simulink model "aerodynamic_model_V1"  (R2025b)
settings: Solver=ode4  StartTime=0.0  StopTime=sim_time  FixedStep=Ts  RelTol=1e-3
InitFcn:
  | % Run initial_main.m first to load Ad,As,Tq_prop,Tq_mass,...
values from neighbouring files (symbols this model uses):
  As = sys_sd.A    [initial_main.m]
  Bs = sys_sd.B    [initial_main.m]
  cg_m = eng.cg_m    [initial_main.m]
  Cs = sys_sd.C    [initial_main.m]
  Ds = sys_sd.D    [initial_main.m]
  DynamicsAndFlexibleStates_IC = Simulink.Bus.createMATLABStruct('DynamicsAndFlexibleStates')    [initial_main.m]
  e_thrust_cruise = eng.e_cruise    [initial_main.m]
  e_thrust_hover = eng.e_hover    [initial_main.m]
  eng_is_tilt = double(eng.is_tilt)    [initial_main.m]
  n_modes = size(Phi, 2)    [aeroelastic.m]    (also in initial_main.m = strips.n_modes)
  p_eng0_m = eng.p_eng_m    [initial_main.m]
  p_kink_m = eng.p_kink_m    [initial_main.m]
  polar_alpha_deg = polar.alpha_deg(:).'    [initial_main.m]
  polar_CD = polar.CD(:).'    [initial_main.m]
  polar_CDp = polar.CDp(:).'    [initial_main.m]
  polar_CL = polar.CL(:).'    [initial_main.m]
  polar_CM = polar.CM(:).'    [initial_main.m]
  R_sb = diag([-1, 1, -1])    [aeroelastic.m]    (also in initial_main.m = eng.R_sb)
  T_m2body = aeroelastic.node_kinematics(Phi, nodes).T_m2body    [initial_main.m]
  Tq_mass = load_maps.Tq_mass    [initial_main.m]
  Tq_prop = load_maps.Tq_prop    [initial_main.m]
  Ts = dt    (= 0.001)    [initial_main.m]
  U = hypot(38.69221536838454, 3.1651981735079)    [initial_main.m]
  v_tail_cant_rad = deg2rad(42)    [initial_main.m]
  W_mass_g = aeroelastic.gravity(nodes, 'g', g).W_mass    [initial_main.m]
  x0_structure = zeros(size(As, 1), 1)    [initial_main.m]
undefined symbols (not defined in the file or in its folder): Ad_v_tail_L, Ad_v_tail_R, Ad_wing_L, Ad_wing_R, alpha_du0_v_tail_L, alpha_du0_v_tail_R, alpha_du0_wing_L, alpha_du0_wing_R, Bd_v_tail_L, Bd_v_tail_R, Bd_wing_L, Bd_wing_R, c_over_2U_v_tail_L, c_over_2U_v_tail_R, c_over_2U_wing_L, c_over_2U_wing_R, Cd_v_tail_L, Cd_v_tail_R, Cd_wing_L, Cd_wing_R, cfd2d_ja, cfd2d_jl, cfd2d_kQ, cfd2d_kT, cfd2d_P1_CEF_X, cfd2d_P1_CEF_Y, cfd2d_P1_CEF_Z, cfd2d_P1_CEM_X, cfd2d_P1_CEM_Y, cfd2d_P1_CEM_Z, cfd2d_P5_CEF_X, cfd2d_P5_CEF_Y, cfd2d_P5_CEF_Z, cfd2d_P5_CEM_X, cfd2d_P5_CEM_Y, cfd2d_P5_CEM_Z, cfd3d_ja, cfd3d_jl, cfd3d_P2_CEF_X, cfd3d_P2_CEF_Y, cfd3d_P2_CEF_Z, cfd3d_P2_CEM_X, cfd3d_P2_CEM_Y, cfd3d_P2_CEM_Z, cfd3d_P6_CEF_X, cfd3d_P6_CEF_Y, cfd3d_P6_CEF_Z, cfd3d_P6_CEM_X, cfd3d_P6_CEM_Y, cfd3d_P6_CEM_Z, cfd3d_pitch, Dd_v_tail_L, Dd_v_tail_R, Dd_wing_L, Dd_wing_R, G_du_v_tail_L, G_du_v_tail_R, G_du_wing_L, G_du_wing_R, magnitude ... (+32)
(part 2 of 2)

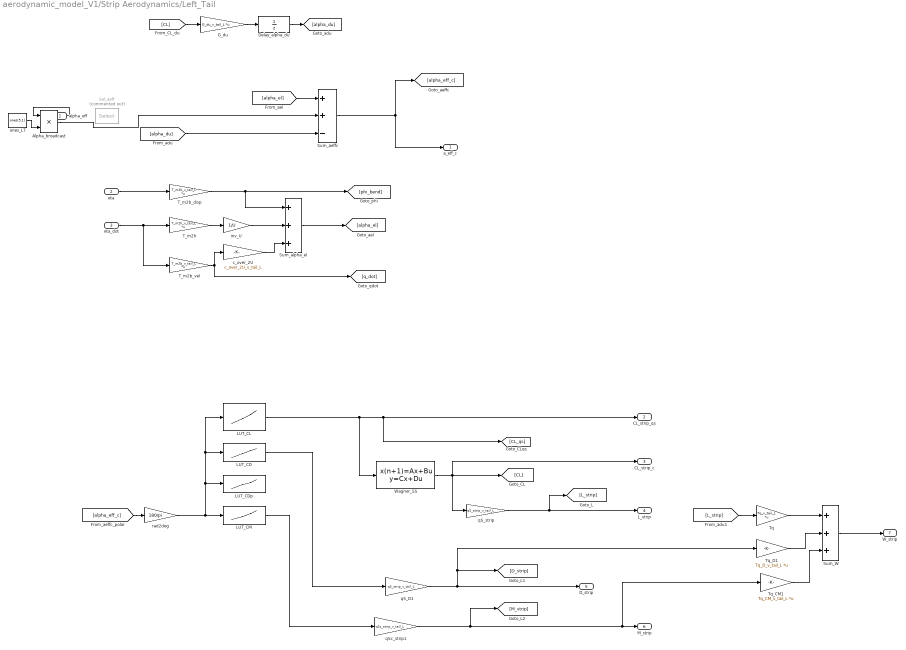
== system aerodynamic_model_V1/Strip Aerodynamics/Left_Tail ==
  alpha_eff : Inport  PortDimensions=1
  eta : Inport  Port=2  PortDimensions=21
  eta_dot : Inport  Port=3  PortDimensions=21
  Alpha_broadcast : Product  Inputs=**
  Delay_alpha_du : UnitDelay  InitialCondition=alpha_du0_v_tail_L  SampleTime=Ts  HasFrameUpgradeWarning=on
  G_du : Gain  Gain=G_du_v_tail_L  Multiplication=Matrix(K*u)
  LUT_CD : Lookup_n-D  NumberOfTableDimensions=1  BreakpointsForDimension1=polar_alpha_deg  BreakpointsForDimension3=[5, 7]  Table=polar_CD  ExtrapMethod=Clip  InternalRulePriority=Speed  RndMeth=Simplest
  LUT_CDp : Lookup_n-D  NumberOfTableDimensions=1  BreakpointsForDimension1=polar_alpha_deg  BreakpointsForDimension3=[5, 7]  Table=polar_CDp  ExtrapMethod=Clip  InternalRulePriority=Speed  RndMeth=Simplest
  LUT_CL : Lookup_n-D  NumberOfTableDimensions=1  BreakpointsForDimension1=polar_alpha_deg  BreakpointsForDimension3=[5, 7]  Table=polar_CL  ExtrapMethod=Clip  InternalRulePriority=Speed  RndMeth=Simplest
  LUT_CM : Lookup_n-D  NumberOfTableDimensions=1  BreakpointsForDimension1=polar_alpha_deg  BreakpointsForDimension3=[5, 7]  Table=polar_CM  ExtrapMethod=Clip  InternalRulePriority=Speed  RndMeth=Simplest
  Sel_aeff : Selector  Commented=on  InputPortWidth=n_strip  IndexOptions=Select all  Indices=idx_v_tail_L  OutputSizes=n_strip_v_tail_L
  Sum_W : Sum  Inputs=+++
  Sum_aeffc : Sum  Inputs=++-
  Sum_alpha_el : Sum  Inputs=+++
  T_m2b_disp : Gain  Gain=T_m2b_v_tail_L  Multiplication=Matrix(K*u)
  T_m2b_vel : Gain  Gain=T_m2b_v_tail_L  Multiplication=Matrix(K*u)
  T_m2h : Gain  Gain=T_m2h_v_tail_L  Multiplication=Matrix(K*u)
  Tq : Gain  Gain=Tq_v_tail_L  Multiplication=Matrix(K*u)
  Tq_CM1 : Gain  Gain=Tq_CM_v_tail_L  Multiplication=Matrix(K*u)
  Tq_D1 : Gain  Gain=Tq_D_v_tail_L  Multiplication=Matrix(K*u)
  Wagner_SS : DiscreteStateSpace  A=Ad_v_tail_L  B=Bd_v_tail_L  C=Cd_v_tail_L  D=Dd_v_tail_L  InitialCondition=x0_wagner_v_tail_L  SampleTime=Ts
  c_over_2U : Gain  Gain=c_over_2U_v_tail_L
  inv_U : Gain  Gain=1/U
  ones_LT : Constant  Value=ones(5,1)
  qS_D1 : Gain  Gain=qS_strip_v_tail_L
  qS_strip : Gain  Gain=qS_strip_v_tail_L
  qSc_strip1 : Gain  Gain=qSc_strip_v_tail_L
  rad2deg : Gain  Gain=180/pi
  a_eff_c : Outport
  CL_strip_qs : Outport  Port=2
  CL_strip_c : Outport  Port=3
  L_strip : Outport  Port=4
  D_strip : Outport  Port=5
  M_strip : Outport  Port=6
  W_strip : Outport  Port=7
  wires:
  rad2deg/1 -> LUT_CL/1, LUT_CD/1, LUT_CDp/1, LUT_CM/1
  Wagner_SS/1 -> [CL], CL_strip_c/1, qS_strip/1
  eta/1 -> T_m2b_disp/1
  Delay_alpha_du/1 -> [alpha_du]
  qS_strip/1 -> L_strip/1, [L_strip]
  LUT_CL/1 -> CL_strip_qs/1, [CL_qs], Wagner_SS/1
  T_m2b_vel/1 -> c_over_2U/1, [q_dot]
  inv_U/1 -> Sum_alpha_el/2
  T_m2b_disp/1 -> Sum_alpha_el/1, [phi_bend]
  G_du/1 -> Delay_alpha_du/1
  c_over_2U/1 -> Sum_alpha_el/3
  Sum_alpha_el/1 -> [alpha_el]
  Sum_aeffc/1 -> a_eff_c/1, [alpha_eff_c]
  [alpha_eff_c] -> rad2deg/1
  T_m2h/1 -> inv_U/1
  eta_dot/1 -> T_m2b_vel/1, T_m2h/1
  LUT_CD/1 -> qS_D1/1
  LUT_CM/1 -> qSc_strip1/1
  [CL] -> G_du/1
  [alpha_el] -> Sum_aeffc/1
  [alpha_du] -> Sum_aeffc/3
  qS_D1/1 -> Tq_D1/1, [D_strip], D_strip/1
  qSc_strip1/1 -> M_strip/1, Tq_CM1/1, [M_strip]
  [L_strip] -> Tq/1
  Tq/1 -> Sum_W/1
  Tq_D1/1 -> Sum_W/2
  Tq_CM1/1 -> Sum_W/3
  Sum_W/1 -> W_strip/1
  alpha_eff/1 -> Alpha_broadcast/1
  ones_LT/1 -> Alpha_broadcast/2
  Alpha_broadcast/1 -> Sum_aeffc/2

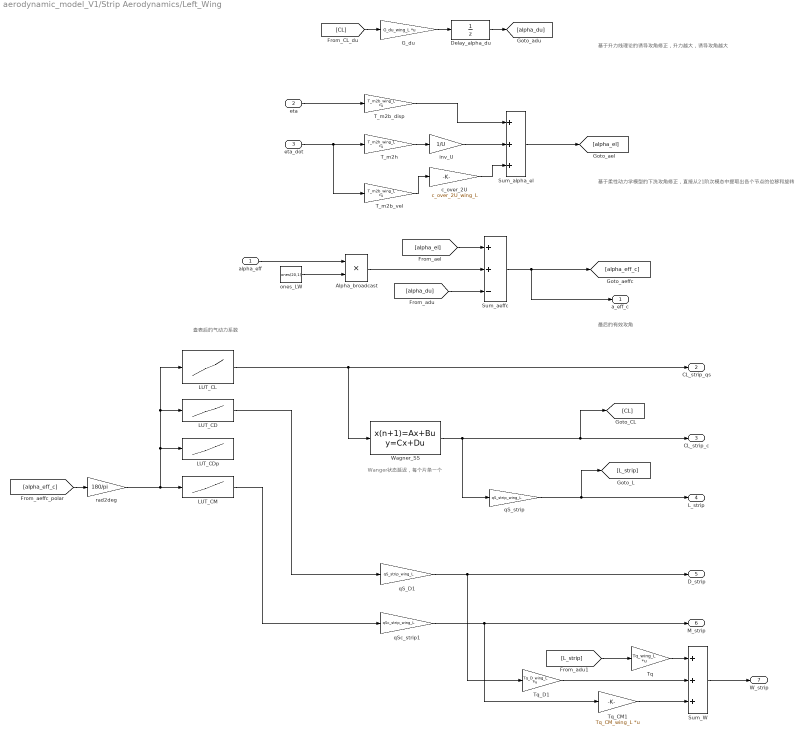
== system aerodynamic_model_V1/Strip Aerodynamics/Left_Wing ==
  note: 基于升力线理论的诱导攻角修正，升力越大，诱导攻角越大
  note: 基于柔性动力学模型的下洗攻角修正，直接从21阶次模态中提取出各个节点的位移和旋转
  note: 最后的有效攻角
  note: 查表后的气动力系数
  note: Wanger状态延迟，每个片条一个
  alpha_eff : Inport  PortDimensions=1
  eta : Inport  Port=2  PortDimensions=21
  eta_dot : Inport  Port=3  PortDimensions=21
  Alpha_broadcast : Product  Inputs=**
  Delay_alpha_du : UnitDelay  InitialCondition=alpha_du0_wing_L  SampleTime=Ts  HasFrameUpgradeWarning=on
  G_du : Gain  Gain=G_du_wing_L  Multiplication=Matrix(K*u)
  LUT_CD : Lookup_n-D  NumberOfTableDimensions=1  BreakpointsForDimension1=polar_alpha_deg  BreakpointsForDimension3=[5, 7]  Table=polar_CD  ExtrapMethod=Clip  InternalRulePriority=Speed  RndMeth=Simplest
  LUT_CDp : Lookup_n-D  NumberOfTableDimensions=1  BreakpointsForDimension1=polar_alpha_deg  BreakpointsForDimension3=[5, 7]  Table=polar_CDp  ExtrapMethod=Clip  InternalRulePriority=Speed  RndMeth=Simplest
  LUT_CL : Lookup_n-D  NumberOfTableDimensions=1  BreakpointsForDimension1=polar_alpha_deg  BreakpointsForDimension3=[5, 7]  Table=polar_CL  ExtrapMethod=Clip  InternalRulePriority=Speed  RndMeth=Simplest
  LUT_CM : Lookup_n-D  NumberOfTableDimensions=1  BreakpointsForDimension1=polar_alpha_deg  BreakpointsForDimension3=[5, 7]  Table=polar_CM  ExtrapMethod=Clip  InternalRulePriority=Speed  RndMeth=Simplest
  Sum_W : Sum  Inputs=+++
  Sum_aeffc : Sum  Inputs=++-
  Sum_alpha_el : Sum  Inputs=+++
  T_m2b_disp : Gain  Gain=T_m2b_wing_L  Multiplication=Matrix(K*u)
  T_m2b_vel : Gain  Gain=T_m2b_wing_L  Multiplication=Matrix(K*u)
  T_m2h : Gain  Gain=T_m2h_wing_L  Multiplication=Matrix(K*u)
  Tq : Gain  Gain=Tq_wing_L  Multiplication=Matrix(K*u)
  Tq_CM1 : Gain  Gain=Tq_CM_wing_L  Multiplication=Matrix(K*u)
  Tq_D1 : Gain  Gain=Tq_D_wing_L  Multiplication=Matrix(K*u)
  Wagner_SS : DiscreteStateSpace  A=Ad_wing_L  B=Bd_wing_L  C=Cd_wing_L  D=Dd_wing_L  InitialCondition=x0_wagner_wing_L  SampleTime=Ts
  c_over_2U : Gain  Gain=c_over_2U_wing_L
  inv_U : Gain  Gain=1/U
  ones_LW : Constant  Value=ones(20,1)
  qS_D1 : Gain  Gain=qS_strip_wing_L
  qS_strip : Gain  Gain=qS_strip_wing_L
  qSc_strip1 : Gain  Gain=qSc_strip_wing_L
  rad2deg : Gain  Gain=180/pi
  a_eff_c : Outport
  CL_strip_qs : Outport  Port=2
  CL_strip_c : Outport  Port=3
  L_strip : Outport  Port=4
  D_strip : Outport  Port=5
  M_strip : Outport  Port=6
  W_strip : Outport  Port=7
  wires:
  rad2deg/1 -> LUT_CL/1, LUT_CD/1, LUT_CDp/1, LUT_CM/1
  Wagner_SS/1 -> [CL], CL_strip_c/1, qS_strip/1
  eta/1 -> T_m2b_disp/1
  Delay_alpha_du/1 -> [alpha_du]
  qS_strip/1 -> L_strip/1, [L_strip]
  LUT_CL/1 -> CL_strip_qs/1, Wagner_SS/1
  T_m2b_vel/1 -> c_over_2U/1
  inv_U/1 -> Sum_alpha_el/2
  T_m2b_disp/1 -> Sum_alpha_el/1
  G_du/1 -> Delay_alpha_du/1
  c_over_2U/1 -> Sum_alpha_el/3
  Sum_alpha_el/1 -> [alpha_el]
  Sum_aeffc/1 -> a_eff_c/1, [alpha_eff_c]
  [alpha_eff_c] -> rad2deg/1
  T_m2h/1 -> inv_U/1
  eta_dot/1 -> T_m2b_vel/1, T_m2h/1
  LUT_CD/1 -> qS_D1/1
  LUT_CM/1 -> qSc_strip1/1
  [CL] -> G_du/1
  [alpha_el] -> Sum_aeffc/1
  [alpha_du] -> Sum_aeffc/3
  qS_D1/1 -> D_strip/1, Tq_D1/1
  qSc_strip1/1 -> M_strip/1, Tq_CM1/1
  [L_strip] -> Tq/1
  Tq/1 -> Sum_W/1
  Tq_D1/1 -> Sum_W/2
  Tq_CM1/1 -> Sum_W/3
  Sum_W/1 -> W_strip/1
  alpha_eff/1 -> Alpha_broadcast/1
  ones_LW/1 -> Alpha_broadcast/2
  Alpha_broadcast/1 -> Sum_aeffc/2

== system aerodynamic_model_V1/Strip Aerodynamics/Local_Alphas ==
  V_b : Inport  PortDimensions=3
  cant : Inport  Port=2  PortDimensions=1
  fcn : MATLAB Function  TreatAsAtomicUnit=on
  a_wr : Outport
  a_wl : Outport  Port=2
  a_tr : Outport  Port=3
  a_tl : Outport  Port=4
  wires:
  V_b/1 -> fcn/1(V_b)
  cant/1 -> fcn/2(cant)
  fcn/1(a_wr) -> a_wr/1
  fcn/2(a_wl) -> a_wl/1
  fcn/3(a_tr) -> a_tr/1
  fcn/4(a_tl) -> a_tl/1

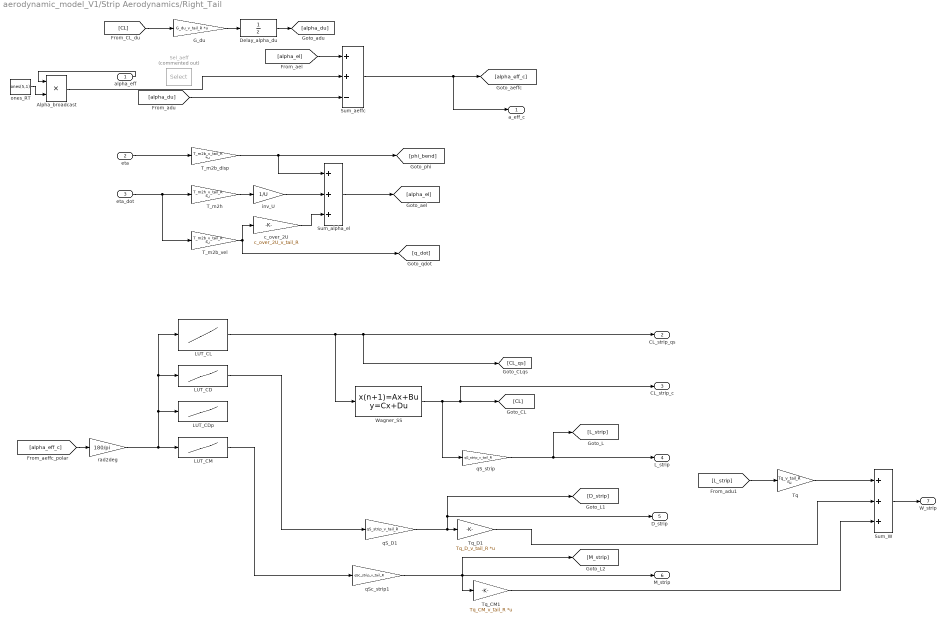
== system aerodynamic_model_V1/Strip Aerodynamics/Right_Tail ==
  alpha_eff : Inport  PortDimensions=1
  eta : Inport  Port=2  PortDimensions=21
  eta_dot : Inport  Port=3  PortDimensions=21
  Alpha_broadcast : Product  Inputs=**
  Delay_alpha_du : UnitDelay  InitialCondition=alpha_du0_v_tail_R  SampleTime=Ts  HasFrameUpgradeWarning=on
  G_du : Gain  Gain=G_du_v_tail_R  Multiplication=Matrix(K*u)
  LUT_CD : Lookup_n-D  NumberOfTableDimensions=1  BreakpointsForDimension1=polar_alpha_deg  BreakpointsForDimension3=[5, 7]  Table=polar_CD  ExtrapMethod=Clip  InternalRulePriority=Speed  RndMeth=Simplest
  LUT_CDp : Lookup_n-D  NumberOfTableDimensions=1  BreakpointsForDimension1=polar_alpha_deg  BreakpointsForDimension3=[5, 7]  Table=polar_CDp  ExtrapMethod=Clip  InternalRulePriority=Speed  RndMeth=Simplest
  LUT_CL : Lookup_n-D  NumberOfTableDimensions=1  BreakpointsForDimension1=polar_alpha_deg  BreakpointsForDimension3=[5, 7]  Table=polar_CL  ExtrapMethod=Clip  InternalRulePriority=Speed  RndMeth=Simplest
  LUT_CM : Lookup_n-D  NumberOfTableDimensions=1  BreakpointsForDimension1=polar_alpha_deg  BreakpointsForDimension3=[5, 7]  Table=polar_CM  ExtrapMethod=Clip  InternalRulePriority=Speed  RndMeth=Simplest
  Sel_aeff : Selector  Commented=on  InputPortWidth=n_strip  IndexOptions=Select all  Indices=idx_v_tail_R  OutputSizes=n_strip_v_tail_R
  Sum_W : Sum  Inputs=+++
  Sum_aeffc : Sum  Inputs=++-
  Sum_alpha_el : Sum  Inputs=+++
  T_m2b_disp : Gain  Gain=T_m2b_v_tail_R  Multiplication=Matrix(K*u)
  T_m2b_vel : Gain  Gain=T_m2b_v_tail_R  Multiplication=Matrix(K*u)
  T_m2h : Gain  Gain=T_m2h_v_tail_R  Multiplication=Matrix(K*u)
  Tq : Gain  Gain=Tq_v_tail_R  Multiplication=Matrix(K*u)
  Tq_CM1 : Gain  Gain=Tq_CM_v_tail_R  Multiplication=Matrix(K*u)
  Tq_D1 : Gain  Gain=Tq_D_v_tail_R  Multiplication=Matrix(K*u)
  Wagner_SS : DiscreteStateSpace  A=Ad_v_tail_R  B=Bd_v_tail_R  C=Cd_v_tail_R  D=Dd_v_tail_R  InitialCondition=x0_wagner_v_tail_R  SampleTime=Ts
  c_over_2U : Gain  Gain=c_over_2U_v_tail_R
  inv_U : Gain  Gain=1/U
  ones_RT : Constant  Value=ones(5,1)
  qS_D1 : Gain  Gain=qS_strip_v_tail_R
  qS_strip : Gain  Gain=qS_strip_v_tail_R
  qSc_strip1 : Gain  Gain=qSc_strip_v_tail_R
  rad2deg : Gain  Gain=180/pi
  a_eff_c : Outport
  CL_strip_qs : Outport  Port=2
  CL_strip_c : Outport  Port=3
  L_strip : Outport  Port=4
  D_strip : Outport  Port=5
  M_strip : Outport  Port=6
  W_strip : Outport  Port=7
  wires:
  rad2deg/1 -> LUT_CL/1, LUT_CD/1, LUT_CDp/1, LUT_CM/1
  Wagner_SS/1 -> CL_strip_c/1, [CL], qS_strip/1
  eta/1 -> T_m2b_disp/1
  Delay_alpha_du/1 -> [alpha_du]
  qS_strip/1 -> L_strip/1, [L_strip]
  LUT_CL/1 -> CL_strip_qs/1, [CL_qs], Wagner_SS/1
  T_m2b_vel/1 -> c_over_2U/1, [q_dot]
  inv_U/1 -> Sum_alpha_el/2
  T_m2b_disp/1 -> Sum_alpha_el/1, [phi_bend]
  G_du/1 -> Delay_alpha_du/1
  c_over_2U/1 -> Sum_alpha_el/3
  Sum_alpha_el/1 -> [alpha_el]
  Sum_aeffc/1 -> a_eff_c/1, [alpha_eff_c]
  [alpha_eff_c] -> rad2deg/1
  T_m2h/1 -> inv_U/1
  eta_dot/1 -> T_m2b_vel/1, T_m2h/1
  LUT_CD/1 -> qS_D1/1
  LUT_CM/1 -> qSc_strip1/1
  [CL] -> G_du/1
  [alpha_el] -> Sum_aeffc/1
  [alpha_du] -> Sum_aeffc/3
  qS_D1/1 -> D_strip/1, [D_strip], Tq_D1/1
  qSc_strip1/1 -> [M_strip], M_strip/1, Tq_CM1/1
  [L_strip] -> Tq/1
  Tq/1 -> Sum_W/1
  Tq_D1/1 -> Sum_W/2
  Tq_CM1/1 -> Sum_W/3
  Sum_W/1 -> W_strip/1
  alpha_eff/1 -> Alpha_broadcast/1
  ones_RT/1 -> Alpha_broadcast/2
  Alpha_broadcast/1 -> Sum_aeffc/2

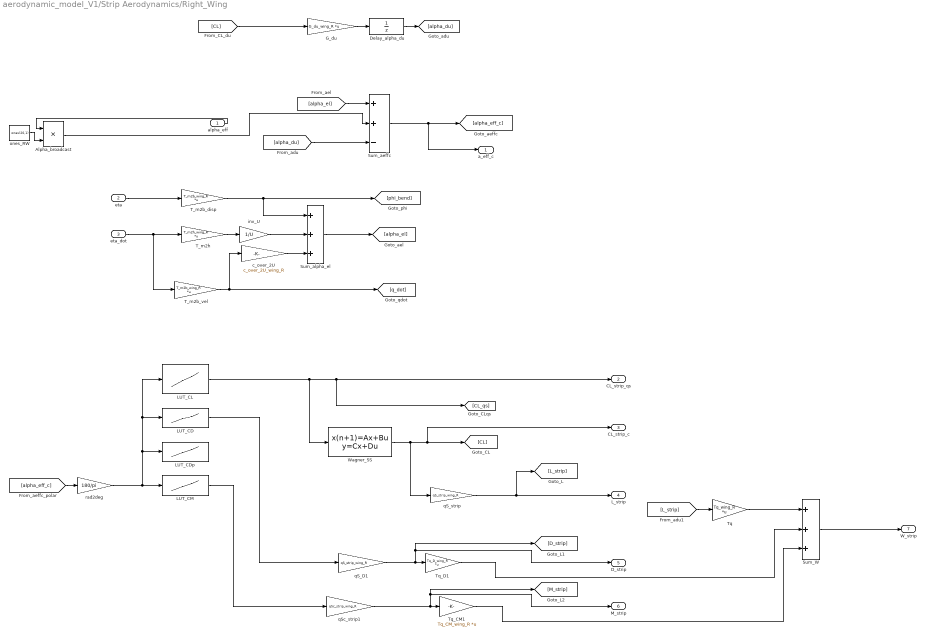
== system aerodynamic_model_V1/Strip Aerodynamics/Right_Wing ==
  alpha_eff : Inport  PortDimensions=1
  eta : Inport  Port=2  PortDimensions=21
  eta_dot : Inport  Port=3  PortDimensions=21
  Alpha_broadcast : Product  Inputs=**
  Delay_alpha_du : UnitDelay  InitialCondition=alpha_du0_wing_R  SampleTime=Ts  HasFrameUpgradeWarning=on
  G_du : Gain  Gain=G_du_wing_R  Multiplication=Matrix(K*u)
  LUT_CD : Lookup_n-D  NumberOfTableDimensions=1  BreakpointsForDimension1=polar_alpha_deg  BreakpointsForDimension3=[5, 7]  Table=polar_CD  ExtrapMethod=Clip  InternalRulePriority=Speed  RndMeth=Simplest
  LUT_CDp : Lookup_n-D  NumberOfTableDimensions=1  BreakpointsForDimension1=polar_alpha_deg  BreakpointsForDimension3=[5, 7]  Table=polar_CDp  ExtrapMethod=Clip  InternalRulePriority=Speed  RndMeth=Simplest
  LUT_CL : Lookup_n-D  NumberOfTableDimensions=1  BreakpointsForDimension1=polar_alpha_deg  BreakpointsForDimension3=[5, 7]  Table=polar_CL  ExtrapMethod=Clip  InternalRulePriority=Speed  RndMeth=Simplest
  LUT_CM : Lookup_n-D  NumberOfTableDimensions=1  BreakpointsForDimension1=polar_alpha_deg  BreakpointsForDimension3=[5, 7]  Table=polar_CM  ExtrapMethod=Clip  InternalRulePriority=Speed  RndMeth=Simplest
  Sum_W : Sum  Inputs=+++
  Sum_aeffc : Sum  Inputs=++-
  Sum_alpha_el : Sum  Inputs=+++
  T_m2b_disp : Gain  Gain=T_m2b_wing_R  Multiplication=Matrix(K*u)
  T_m2b_vel : Gain  Gain=T_m2b_wing_R  Multiplication=Matrix(K*u)
  T_m2h : Gain  Gain=T_m2h_wing_R  Multiplication=Matrix(K*u)
  Tq : Gain  Gain=Tq_wing_R  Multiplication=Matrix(K*u)
  Tq_CM1 : Gain  Gain=Tq_CM_wing_R  Multiplication=Matrix(K*u)
  Tq_D1 : Gain  Gain=Tq_D_wing_R  Multiplication=Matrix(K*u)
  Wagner_SS : DiscreteStateSpace  A=Ad_wing_R  B=Bd_wing_R  C=Cd_wing_R  D=Dd_wing_R  InitialCondition=x0_wagner_wing_R  SampleTime=Ts
  c_over_2U : Gain  Gain=c_over_2U_wing_R
  inv_U : Gain  Gain=1/U
  ones_RW : Constant  Value=ones(20,1)
  qS_D1 : Gain  Gain=qS_strip_wing_R
  qS_strip : Gain  Gain=qS_strip_wing_R
  qSc_strip1 : Gain  Gain=qSc_strip_wing_R
  rad2deg : Gain  Gain=180/pi
  a_eff_c : Outport
  CL_strip_qs : Outport  Port=2
  CL_strip_c : Outport  Port=3
  L_strip : Outport  Port=4
  D_strip : Outport  Port=5
  M_strip : Outport  Port=6
  W_strip : Outport  Port=7
  wires:
  rad2deg/1 -> LUT_CL/1, LUT_CD/1, LUT_CDp/1, LUT_CM/1
  Wagner_SS/1 -> CL_strip_c/1, [CL], qS_strip/1
  eta/1 -> T_m2b_disp/1
  Delay_alpha_du/1 -> [alpha_du]
  qS_strip/1 -> L_strip/1, [L_strip]
  LUT_CL/1 -> CL_strip_qs/1, [CL_qs], Wagner_SS/1
  T_m2b_vel/1 -> c_over_2U/1, [q_dot]
  inv_U/1 -> Sum_alpha_el/2
  T_m2b_disp/1 -> Sum_alpha_el/1, [phi_bend]
  G_du/1 -> Delay_alpha_du/1
  c_over_2U/1 -> Sum_alpha_el/3
  Sum_alpha_el/1 -> [alpha_el]
  Sum_aeffc/1 -> a_eff_c/1, [alpha_eff_c]
  [alpha_eff_c] -> rad2deg/1
  T_m2h/1 -> inv_U/1
  eta_dot/1 -> T_m2b_vel/1, T_m2h/1
  LUT_CD/1 -> qS_D1/1
  LUT_CM/1 -> qSc_strip1/1
  [CL] -> G_du/1
  [alpha_el] -> Sum_aeffc/1
  [alpha_du] -> Sum_aeffc/3
  qS_D1/1 -> D_strip/1, [D_strip], Tq_D1/1
  qSc_strip1/1 -> M_strip/1, [M_strip], Tq_CM1/1
  [L_strip] -> Tq/1
  Tq/1 -> Sum_W/1
  Tq_D1/1 -> Sum_W/2
  Tq_CM1/1 -> Sum_W/3
  Sum_W/1 -> W_strip/1
  alpha_eff/1 -> Alpha_broadcast/1
  ones_RW/1 -> Alpha_broadcast/2
  Alpha_broadcast/1 -> Sum_aeffc/2

== matlab function aerodynamic_model_V1/Propulsion Dynamics/MATLAB Function ==
  data: Lambda1 input; Lambda2 input; F_mach input; M_mach input; Fq input; Hover1 output; Mq input; Tilt2 output; Tilt3 output; Hover4 output; Hover5 output; Tilt6 output; Tilt7 output; Hover8 output
function [Hover1,Tilt2,Tilt3,Hover4,Hover5,Tilt6,Tilt7,Hover8] = fcn(Lambda1, Lambda2, F_mach, M_mach, Fq, Mq)
L1 = Lambda1(:); L2 = Lambda2(:); Fm = F_mach(:); Mm = M_mach(:);
Fq = Fq(:); Mq = Mq(:);
Hover1 = [L1(1); L2(1); Fm(1); Mm(1); Fq(1); Mq(1)];
Tilt2  = [L1(2); L2(2); Fm(2); Mm(2); Fq(2); Mq(2)];
Tilt3  = [L1(3); L2(3); Fm(3); Mm(3); Fq(3); Mq(3)];
Hover4 = [L1(4); L2(4); Fm(4); Mm(4); Fq(4); Mq(4)];
Hover5 = [L1(5); L2(5); Fm(5); Mm(5); Fq(5); Mq(5)];
Tilt6  = [L1(6); L2(6); Fm(6); Mm(6); Fq(6); Mq(6)];
Tilt7  = [L1(7); L2(7); Fm(7); Mm(7); Fq(7); Mq(7)];
Hover8 = [L1(8); L2(8); Fm(8); Mm(8); Fq(8); Mq(8)];

== matlab function aerodynamic_model_V1/Propulsion Dynamics/Coord_Struct2Body/engine_struct_to_body ==
  data: e_s input; e_b output; p_eng input; p_kink input; e_hinge input; cg input; R_sb input; r_eng_b output; r_stub_b output; e_hinge_b output
function [e_b, r_eng_b, r_stub_b, e_hinge_b] = fcn(e_s, p_eng, p_kink, e_hinge, cg, R_sb)
[e_b, r_eng_b, r_stub_b, e_hinge_b] = engine_struct_to_body(e_s, p_eng, p_kink, e_hinge, cg, R_sb);

== matlab function aerodynamic_model_V1/Propulsion Dynamics/Stub_Pose/engine_stub_pose ==
  data: tilt input; e_s output; e_cruise input; e_hover input; p_kink input; p_eng0 input; is_tilt input; p_eng output; r_stub output; e_hinge output
function [e_s, p_eng, r_stub, e_hinge] = fcn(tilt, e_cruise, e_hover, p_kink, p_eng0, is_tilt)
[e_s, p_eng, r_stub, e_hinge] = engine_stub_pose(tilt, e_cruise, e_hover, p_kink, p_eng0, is_tilt);

== matlab function aerodynamic_model_V1/Propulsion Dynamics/Pack_Wrench/engine_pack_wrenches ==
  data: FM input; W_prop output; e_s input; p_eng input; p_eng0 input; C9 input; R_sb input
function W_prop = fcn(FM, e_s, p_eng, p_eng0, C9, R_sb)
W_prop = engine_pack_wrenches(FM, e_s, p_eng, p_eng0, C9, R_sb);

== matlab function aerodynamic_model_V1/Propulsion Dynamics/Point_Velocity/engine_point_velocity ==
  data: V_b input; V_pt output; omega_b input; r_eng_b input; r_stub_b input; e_hinge_b input; tilt_rate input
function V_pt = fcn(V_b, omega_b, r_eng_b, r_stub_b, e_hinge_b, tilt_rate)
V_pt = engine_point_velocity(V_b, omega_b, r_eng_b, r_stub_b, e_hinge_b, tilt_rate);

== matlab function aerodynamic_model_V1/Propulsion Dynamics/engine_dcm_body_to_eng ==
  data: e_b input; C9 output
function C9 = fcn(e_b)
C9 = engine_dcm_body_to_eng(e_b);

== matlab function aerodynamic_model_V1/Propulsion Dynamics/Aero_Angles/engine_alpha_beta ==
  data: C9 input; alpha output; V_pt input; beta output; Va output; Vl output
function [alpha, beta,Va,Vl] = fcn(C9, V_pt)
[alpha, beta,Va,Vl] = engine_alpha_beta(C9, V_pt);

== matlab function aerodynamic_model_V1/Strip Aerodynamics/Local_Alphas/fcn ==
  data: V_b input; a_wr output; cant input; a_wl output; a_tr output; a_tl output
function [a_wr, a_wl, a_tr, a_tl] = fcn(V_b, cant)
V_b = V_b(:);
if numel(V_b)~=3 || norm(V_b)<1e-6
  a_wr=0; a_wl=0; a_tr=0; a_tl=0; return;
end
Vs = diag([-1,1,-1]) * V_b;
ec = [1;0;0];
sG = sin(cant); cG = cos(cant);
a_wr = atan2(-dot([0;0;1],Vs), -dot(ec,Vs));
a_wl = a_wr;
a_tr = atan2(-dot([0;-sG;cG],Vs), -dot(ec,Vs));
a_tl = atan2(-dot([0; sG;cG],Vs), -dot(ec,Vs));
